simulink model "MecanumAndObjectTrackingModel"  (R2019b)
settings: Solver=VariableStepAuto  StartTime=0.0  StopTime=10.0  RelTol=1e-3
undefined symbols (not defined in the file): objLabel, objX, objY, sampleTime, targetLabel
libraries: mobileRoboticsLib x8
settings Model: Creator=spenc  LastModifiedBy=spenc

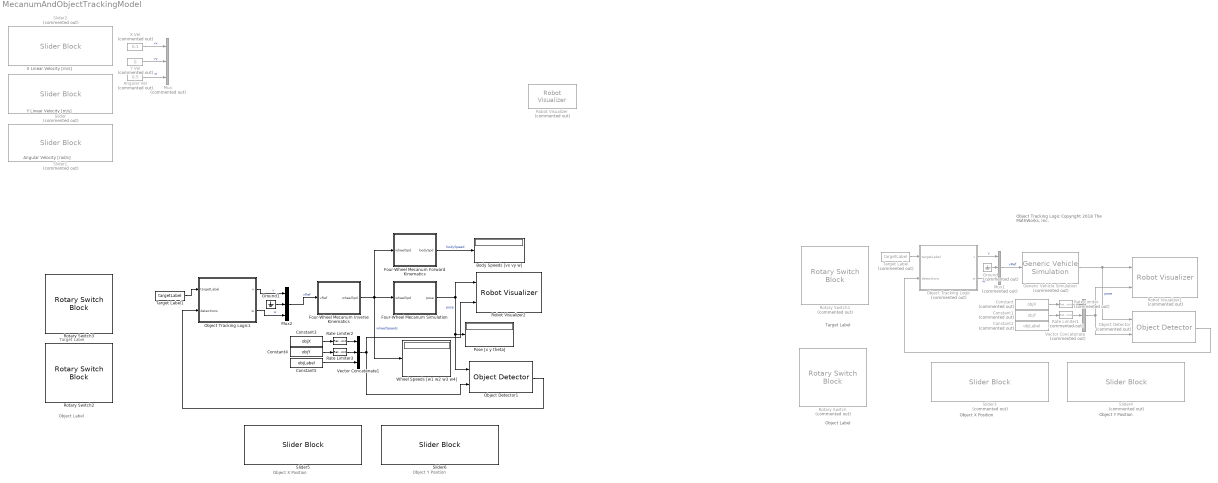
== system MecanumAndObjectTrackingModel ==
  note: Y Linear Velocity [m/s]
  note: Angular Velocity [rad/s]
  note: X Linear Velocity [m/s]
  note: Object X Position
  note: Object Tracking Logic
      |
      | Copyright 2018 The MathWorks, Inc.
  note: Target Label
  note: Object Y Position
  note: Object Label
  note: Object Label
  note: Target Label
  note: Object Y Position
  note: Object X Position
  Angular Vel : Constant  Commented=on  Value=0.5
  Body Speeds [vx vy w] : Display
  Constant : Constant  Commented=on  Value=objX
  Constant1 : Constant  Commented=on  Value=objY
  Constant2 : Constant  Commented=on  Value=objLabel
  Constant3 : Constant  Value=objX
  Constant4 : Constant  Value=objY
  Constant5 : Constant  Value=objLabel
  Four-Wheel Mecanum Forward Kinematics : Subsystem  AncestorBlock=mobileRoboticsLib/Kinematic Models/Four-Wheel Mecanum/Four-Wheel Mecanum Forward Kinematics  mask(Four-Wheel Mecanum Forward Kinematics){wheelRadius=0.1, wheelBase=0.535, wheelTrack=0.459}
      mask prompts: wheelRadius "Wheel Radius [m]"; wheelBase "Wheelbase [m]"; wheelTrack "Track [m]"
      mask help:
      | Calculates the forward kinematics for a four-wheeled vehicle with Mecanum wheels.
      |
      | Input: Wheel speeds [w1; w2; w3; w4] (rad/s)
      |
      | Output: Vehicle velocities [vx; vy; w] in body coordinates (m/s, m/s, and rad/s)
      mask Help: web('matlab:edit mrsDocFourWheelMecanum')
  Four-Wheel Mecanum Inverse Kinematics : Subsystem  AncestorBlock=mobileRoboticsLib/Kinematic Models/Four-Wheel Mecanum/Four-Wheel Mecanum Inverse Kinematics  mask(Four-Wheel Mecanum Inverse Kinematics){wheelRadius=0.1, wheelBase=0.535, wheelTrack=0.459}
      mask prompts: wheelRadius "Wheel Radius [m]"; wheelBase "Wheelbase [m]"; wheelTrack "Track [m]"
      mask help:
      | Calculates the inverse kinematics for a four-wheeled vehicle with Mecanum wheels.
      |
      | Input: Vehicle velocities [vx; vy; w] in body coordinates (m/s, m/s, and rad/s)
      |
      | Output: Wheel speeds [w1; w2; w3; w4] (rad/s)
      mask Help: web('matlab:edit mrsDocFourWheelMecanum')
  Four-Wheel Mecanum Simulation : Subsystem  AncestorBlock=mobileRoboticsLib/Kinematic Models/Four-Wheel Mecanum/Four-Wheel Mecanum Simulation  mask(Four-Wheel Mecanum Simulation){wheelRadius=0.1, wheelBase=0.535, wheelTrack=0.459, initX=0, initY=0, initAngle=0, Ts=0.05}
      mask prompts: wheelRadius "Wheel Radius [m]"; wheelBase "Wheelbase [m]"; wheelTrack "Track [m]"; initX "Initial X Position [m]"; initY "Initial Y Position [m]"; initAngle "Initial Angle [rad]"; Ts "Sample Time"
      mask help:
      | Simulates the kinematics of a four-wheeled vehicle with Mecanum wheels, from a specified initial pose.
      |
      | Input: Wheel speeds [w1; w2; w3; w4] (rad/s)
      |
      | Output: Pose [x; y; theta], in m, m, and rad
      |
      | Set the Sample Time parameter to 0 for continuous-time simulation, or a positive number for discrete-time simulation.
      mask Help: web('matlab:edit mrsDocFourWheelMecanum')
      mask Callback Ts:
      | Ts = evalin('base',get_param(gcb,'Ts'));
      | blk = [gcb '/Generic Robot Simulation/Velocity Integrator'];
      | if Ts > 0
      |     set_param(blk,'OverrideUsingVariant','mode==2');
      | else
      |     set_param(blk,'OverrideUsingVariant','mode==1');
      | end
  Generic Vehicle Simulation : mobileRoboticsLib/Utilities/Generic Vehicle Simulation  Commented=on  initX=2  initY=3  initAngle=0  Ts=sampleTime
      settings: SourceProductName=Mobile Robotics Simulation Library
  Ground : Ground  Commented=on
  Ground1 : Ground
  Mux : Mux  Commented=on  Inputs=3
  Mux1 : Mux  Commented=on  Inputs=3
  Mux2 : Mux  Inputs=3
  Object Detector : mobileRoboticsLib/Environments/Object Detector  Commented=on  mapName=map  sensorOffset=objDetectorOffset  sensorAngle=objDetectorAngle  fieldOfView=objDetectorFOV  maxRange=objDetectorRange  maxDetections=objDetectorMaxHits  sampleTime=-1
      settings: SourceProductName=Ground Vehicles Library
  Object Detector1 : mobileRoboticsLib/Environments/Object Detector  mapName=map  sensorOffset=[0,0]  sensorAngle=0  fieldOfView=pi/4  maxRange=5  maxDetections=3  sampleTime=0.05
      settings: SourceProductName=Ground Vehicles Library
  Object Tracking Logic : Stateflow chart  Commented=on  TreatAsAtomicUnit=on
  Object Tracking Logic1 : Stateflow chart  TreatAsAtomicUnit=on
  Pose [x y theta] : Display
  Rate Limiter : RateLimiter  Commented=on  SampleTimeMode=inherited  InitialCondition=objX
  Rate Limiter1 : RateLimiter  Commented=on  SampleTimeMode=inherited  InitialCondition=objX
  Rate Limiter2 : RateLimiter  SampleTimeMode=inherited  InitialCondition=objX
  Rate Limiter3 : RateLimiter  SampleTimeMode=inherited  InitialCondition=objX
  Robot Visualizer : mobileRoboticsLib/Environments/Robot Visualizer  Priority=99  Commented=on  robotRadius=0  showTrajectory=on  hasWaypoints=off  hasLidar=off  sensorOffset=[ 0 0 ]  scanAngles=scanAngles  hasObjDetector=off  objDetectorOffset=[ 0, 0 ]  objDetectorAngle=0  objDetectorFOV=pi/4  objDetectorMaxRange=5  objectColors=[ 1, 0, 0; 0, 1, 0; 0, 0, 1 ]  objectMarkers=s
      settings: SourceProductName=Ground Vehicles Library
  Robot Visualizer1 : mobileRoboticsLib/Environments/Robot Visualizer  Priority=99  Commented=on  robotRadius=0  mapName=map  showTrajectory=on  hasWaypoints=off  hasLidar=off  sensorOffset=[ 0 0 ]  scanAngles=0  hasObjDetector=on  objDetectorOffset=objDetectorOffset  objDetectorAngle=objDetectorAngle  objDetectorFOV=objDetectorFOV  objDetectorMaxRange=objDetectorRange  objectColors=objDetectorColors  objectMarkers=s
      settings: SourceProductName=Ground Vehicles Library
  Robot Visualizer2 : mobileRoboticsLib/Environments/Robot Visualizer  Priority=99  robotRadius=0.5  mapName=map  showTrajectory=on  hasWaypoints=off  hasLidar=off  sensorOffset=[ 0 0 ]  scanAngles=0  hasObjDetector=on  objDetectorOffset=[0,0]  objDetectorAngle=[-pi/4,0,pi/4]  objDetectorFOV=pi/4  objDetectorMaxRange=5  objectColors=eye(3,3)  objectMarkers=s
      settings: SourceProductName=Ground Vehicles Library
  Rotary Switch : RotarySwitchBlock  Commented=on  LabelPosition=Hide
      settings: Values={{'RED', 'GREEN', 'BLUE'}, [1 2 3]}
  Rotary Switch1 : RotarySwitchBlock  Commented=on  LabelPosition=Hide
      settings: Values={{'RED', 'GREEN', 'BLUE'}, [1 2 3]}
  Rotary Switch2 : RotarySwitchBlock  LabelPosition=Hide
      settings: Values={{'RED', 'GREEN', 'BLUE'}, [1 2 3]}
  Rotary Switch3 : RotarySwitchBlock  LabelPosition=Hide
      settings: Values={{'RED', 'GREEN', 'BLUE'}, [1 2 3]}
  Slider : SliderBlock  Commented=on  ScaleMin=-1  ScaleMax=1  TickInterval=0.25
  Slider1 : SliderBlock  Commented=on  ScaleMin=-1.5  ScaleMax=1.5
  Slider2 : SliderBlock  Commented=on  ScaleMin=-1  ScaleMax=1  TickInterval=0.25
  Slider3 : SliderBlock  Commented=on  ScaleMax=13
  Slider4 : SliderBlock  Commented=on  ScaleMax=13
  Slider5 : SliderBlock  ScaleMax=13
  Slider6 : SliderBlock  ScaleMax=13
  Target Label : Constant  Commented=on  Value=targetLabel
  Target Label1 : Constant  Value=targetLabel
  Vector Concatenate : Concatenate  Commented=on  NumInputs=3  Mode=Multidimensional array  ConcatenateDimension=2
  Vector Concatenate1 : Concatenate  NumInputs=3  Mode=Multidimensional array  ConcatenateDimension=2
  Wheel Speeds [w1 w2 w3 w4] : Display
  X Vel : Constant  Commented=on  Value=0.1
  Y Vel : Constant  Commented=on  Value=0
  wires:
  Y Vel/1 -> Mux/2  "vy"
  Four-Wheel Mecanum Forward Kinematics/1(bodySpd) -> Body Speeds [vx vy w]/1  "bodySpeed"
  Four-Wheel Mecanum Simulation/1(pose) -> Robot Visualizer2/1, Object Detector1/1, Pose [x y theta]/1  "pose"
  Four-Wheel Mecanum Inverse Kinematics/1(wheelSpd) -> Four-Wheel Mecanum Forward Kinematics/1(wheelSpd), Four-Wheel Mecanum Simulation/1(wheelSpd), Wheel Speeds [w1 w2 w3 w4]/1  "wheelSpeeds"
  Angular Vel/1 -> Mux/3  "w"
  X Vel/1 -> Mux/1  "vx"
  Ground/1 -> Mux1/2
  Rate Limiter1/1 -> Vector Concatenate/2
  Target Label/1 -> Object Tracking Logic/1(targetLabel)
  Rate Limiter/1 -> Vector Concatenate/1
  Generic Vehicle Simulation/1 -> Object Detector/1, Robot Visualizer1/1  "pose"
  Object Tracking Logic/2(w) -> Mux1/3  "w"
  Vector Concatenate/1 -> Object Detector/2, Robot Visualizer1/2
  Object Tracking Logic/1(v) -> Mux1/1  "v"
  Object Detector/1 -> Object Tracking Logic/2(detections)
  Constant/1 -> Rate Limiter/1
  Mux1/1 -> Generic Vehicle Simulation/1  "vRef"
  Constant2/1 -> Vector Concatenate/3
  Constant1/1 -> Rate Limiter1/1
  Mux2/1 -> Four-Wheel Mecanum Inverse Kinematics/1(vRef)  "vRef"
  Object Detector1/1 -> Object Tracking Logic1/2(detections)
  Object Tracking Logic1/2(w) -> Mux2/3  "w"
  Target Label1/1 -> Object Tracking Logic1/1(targetLabel)
  Ground1/1 -> Mux2/2
  Object Tracking Logic1/1(v) -> Mux2/1  "v"
  Constant4/1 -> Rate Limiter3/1
  Constant5/1 -> Vector Concatenate1/3
  Constant3/1 -> Rate Limiter2/1
  Rate Limiter2/1 -> Vector Concatenate1/1
  Rate Limiter3/1 -> Vector Concatenate1/2
  Vector Concatenate1/1 -> Object Detector1/2, Robot Visualizer2/2

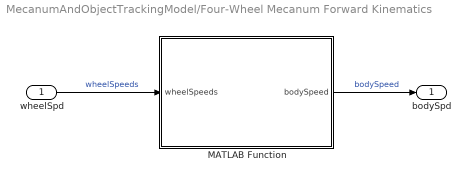
== system MecanumAndObjectTrackingModel/Four-Wheel Mecanum Forward Kinematics ==
  wheelSpd : Inport
  MATLAB Function : MATLAB Function  TreatAsAtomicUnit=on
  bodySpd : Outport  VectorParamsAs1DForOutWhenUnconnected=off
  wires:
  wheelSpd/1 -> MATLAB Function/1(wheelSpeeds)  "wheelSpeeds"
  MATLAB Function/1(bodySpeed) -> bodySpd/1  "bodySpeed"

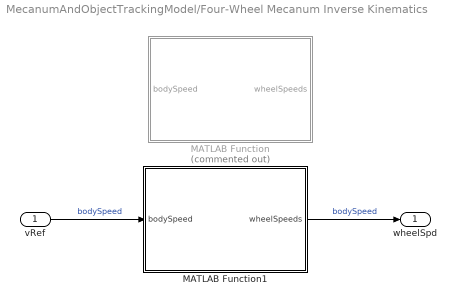
== system MecanumAndObjectTrackingModel/Four-Wheel Mecanum Inverse Kinematics ==
  vRef : Inport
  MATLAB Function : MATLAB Function  Commented=on  TreatAsAtomicUnit=on
  MATLAB Function1 : MATLAB Function  TreatAsAtomicUnit=on
  wheelSpd : Outport  VectorParamsAs1DForOutWhenUnconnected=off
  wires:
  vRef/1 -> MATLAB Function1/1(bodySpeed)  "bodySpeed"
  MATLAB Function1/1(wheelSpeeds) -> wheelSpd/1  "bodySpeed"

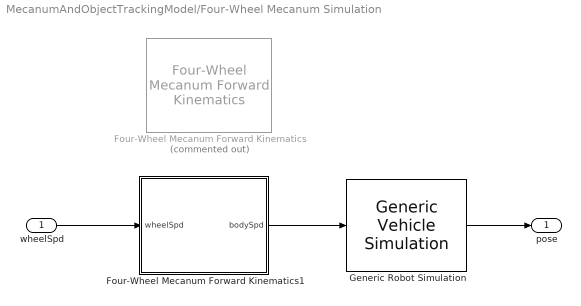
== system MecanumAndObjectTrackingModel/Four-Wheel Mecanum Simulation ==
  wheelSpd : Inport
  Four-Wheel Mecanum Forward Kinematics : mobileRoboticsLib/Kinematic Models/Four-Wheel Mecanum/Four-Wheel Mecanum Forward Kinematics  Commented=on  wheelRadius=0.1  wheelBase=0.535  wheelTrack=0.459
      settings: SourceProductName=Mobile Robotics Simulation Toolbox
  Four-Wheel Mecanum Forward Kinematics1 : Subsystem  AncestorBlock=mobileRoboticsLib/Kinematic Models/Four-Wheel Mecanum/Four-Wheel Mecanum Forward Kinematics  mask(Four-Wheel Mecanum Forward Kinematics){wheelRadius=0.1, wheelBase=0.535, wheelTrack=0.459}
      mask prompts: wheelRadius "Wheel Radius [m]"; wheelBase "Wheelbase [m]"; wheelTrack "Track [m]"
      mask help:
      | Calculates the forward kinematics for a four-wheeled vehicle with Mecanum wheels.
      |
      | Input: Wheel speeds [w1; w2; w3; w4] (rad/s)
      |
      | Output: Vehicle velocities [vx; vy; w] in body coordinates (m/s, m/s, and rad/s)
      mask Help: web('matlab:edit mrsDocFourWheelMecanum')
  Generic Robot Simulation : mobileRoboticsLib/Utilities/Generic Vehicle Simulation  initX=initX  initY=initY  initAngle=initAngle  Ts=Ts
      settings: SourceProductName=Mobile Robotics Simulation Toolbox
  pose : Outport  VectorParamsAs1DForOutWhenUnconnected=off
  wires:
  Generic Robot Simulation/1 -> pose/1
  wheelSpd/1 -> Four-Wheel Mecanum Forward Kinematics1/1(wheelSpd)
  Four-Wheel Mecanum Forward Kinematics1/1(bodySpd) -> Generic Robot Simulation/1

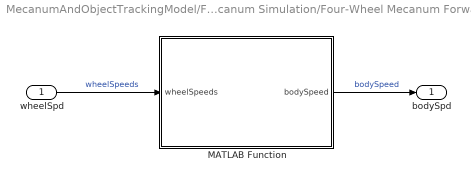
== system MecanumAndObjectTrackingModel/Four-Wheel Mecanum Simulation/Four-Wheel Mecanum Forward Kinematics1 ==
  wheelSpd : Inport
  MATLAB Function : MATLAB Function  TreatAsAtomicUnit=on
  bodySpd : Outport  VectorParamsAs1DForOutWhenUnconnected=off
  wires:
  MATLAB Function/1(bodySpeed) -> bodySpd/1  "bodySpeed"
  wheelSpd/1 -> MATLAB Function/1(wheelSpeeds)  "wheelSpeeds"

== stateflow chart MecanumAndObjectTrackingModel/Object Tracking Logic1 ==
  state TrackObject
    entry, during:
    [range,angle,valid] = findValidObject(targetLabel);
    if valid
    count = 0;
    else
    count = count + 1;
    end
    (default) -> (junction 20)
    TrackObject -> (junction 20) [order 1]
    (junction 20) -> (junction 24) [order 1] : % Set angular speed if
        | % angle outside deadband
        | [abs(angle) > pi/24]
    (junction 20) -> (junction 30) [order 2] : {w = 0;}
    (junction 24) -> (junction 49) : % Proportional
        | % control
        | {w = 1.5*angle;}
    (junction 49) -> (junction 30)
    (junction 30) -> (junction 54)
    (junction 54) -> (junction 56) [order 1] : % Go forward if object is far
        | [range > 1]
    (junction 54) -> (junction 60) [order 2] : {v = 0;}
    (junction 56) -> (junction 58) : {v = 0.5;}
    (junction 58) -> (junction 60)
  state SeekObject
    entry:
    v = 0;
    w = 1;
  (default) -> TrackObject : {
      | count = 0;
      | range = 0;
      | angle = 0;
      | }
  TrackObject -> SeekObject [order 1] : [count > 20]
  SeekObject -> TrackObject : [~isempty(detections)]
  data: dist function_output; ang function_output; flag function_output; label function_input; targetLabel input; detections input size=[objDetectorMaxHits,3]; v output; w output; angle local; range local; count local; valid local
  function [dist,ang,flag] = findValidObject(label):
    | function [dist,ang,flag] = findValidObject(label)
    | % Finds the distance (dist) and angle (ang) of the nearest valid
    | % object detected. If an object is found, the (flag) output is true.
    | 
    | % Initialize
    | flag = false;
    | dist = 0;
    | ang = 0;
    | 
    | if ~isempty(detections)
    |     % Loop through all detections
    |     for idx = 1:size(detections,1)
    |         % If a detection matching the target label is found, 
    |         % return it and set the valid flag to true.
    |         if detections(idx,3) == label
    |             dist = detections(idx,1);
    |             ang  = detections(idx,2);
    |             flag = true;
    |             return; 
    |         end
    |     end
    | end

== matlab function MecanumAndObjectTrackingModel/Four-Wheel Mecanum Inverse Kinematics/MATLAB Function1 ==
  data: bodySpeed input; wheelRadius parameter; wheelSpeeds output; wheelBase parameter; wheelTrack parameter
function wheelSpeeds = fourWheelMecanumInvKin(bodySpeed,wheelRadius,wheelBase,wheelTrack)
    
    % Initialize FourWheelMecanum object
    persistent robot
    if isempty(robot)
        robot = FourWheelMecanum_toolbox(wheelRadius,wheelBase,wheelTrack);
    end
    
    % Run object's inverse kinematics method
    wheelSpeeds = inverseKinematics(robot,bodySpeed);

end

== stateflow chart MecanumAndObjectTrackingModel/Object Tracking Logic ==
  state TrackObject
    entry, during:
    [range,angle,valid] = findValidObject(targetLabel);
    if valid
    count = 0;
    else
    count = count + 1;
    end
    (default) -> (junction 20)
    TrackObject -> (junction 20) [order 1]
    (junction 20) -> (junction 24) [order 1] : % Set angular speed if
        | % angle outside deadband
        | [abs(angle) > pi/24]
    (junction 20) -> (junction 30) [order 2] : {w = 0;}
    (junction 24) -> (junction 49) : % Proportional
        | % control
        | {w = 1.5*angle;}
    (junction 49) -> (junction 30)
    (junction 30) -> (junction 54)
    (junction 54) -> (junction 56) [order 1] : % Go forward if object is far
        | [range > 1]
    (junction 54) -> (junction 60) [order 2] : {v = 0;}
    (junction 56) -> (junction 58) : {v = 0.5;}
    (junction 58) -> (junction 60)
  state SeekObject
    entry:
    v = 0;
    w = 1;
  (default) -> TrackObject : {
      | count = 0;
      | range = 0;
      | angle = 0;
      | }
  TrackObject -> SeekObject [order 1] : [count > 20]
  SeekObject -> TrackObject : [~isempty(detections)]
  data: dist function_output; ang function_output; flag function_output; label function_input; targetLabel input; detections input size=[objDetectorMaxHits,3]; v output; w output; angle local; range local; count local; valid local
  function [dist,ang,flag] = findValidObject(label):
    | function [dist,ang,flag] = findValidObject(label)
    | % Finds the distance (dist) and angle (ang) of the nearest valid
    | % object detected. If an object is found, the (flag) output is true.
    | 
    | % Initialize
    | flag = false;
    | dist = 0;
    | ang = 0;
    | 
    | if ~isempty(detections)
    |     % Loop through all detections
    |     for idx = 1:size(detections,1)
    |         % If a detection matching the target label is found, 
    |         % return it and set the valid flag to true.
    |         if detections(idx,3) == label
    |             dist = detections(idx,1);
    |             ang  = detections(idx,2);
    |             flag = true;
    |             return; 
    |         end
    |     end
    | end

== matlab function MecanumAndObjectTrackingModel/Four-Wheel Mecanum Simulation/Four-Wheel Mecanum Forward Kinematics1/MATLAB Function ==
  settings: updateMethod=DISCRETE
  data: wheelSpeeds input; bodySpeed output; wheelRadius parameter; wheelBase parameter; wheelTrack parameter
function bodySpeed = fourWheelMecanumFwdKin(wheelSpeeds,wheelRadius,wheelBase,wheelTrack)
    
    % Initialize FourWheelMecanum object
    persistent robot
    if isempty(robot)
        robot = FourWheelMecanum_toolbox(wheelRadius,wheelBase,wheelTrack);
    end
    
    % Run object's forward kinematics method
    bodySpeed = forwardKinematics(robot,wheelSpeeds);

end

== matlab function MecanumAndObjectTrackingModel/Four-Wheel Mecanum Forward Kinematics/MATLAB Function ==
  settings: updateMethod=DISCRETE
  data: wheelSpeeds input; bodySpeed output; wheelRadius parameter; wheelBase parameter; wheelTrack parameter
function bodySpeed = fourWheelMecanumFwdKin(wheelSpeeds,wheelRadius,wheelBase,wheelTrack)
    
    % Initialize FourWheelMecanum object
%% 
    persistent robot
    if isempty(robot)
        robot = FourWheelMecanum(wheelRadius,wheelBase,wheelTrack);
    end
    
    % Run object's forward kinematics method
    bodySpeed = forwardKinematics(robot,wheelSpeeds);

end

== matlab function MecanumAndObjectTrackingModel/Four-Wheel Mecanum Inverse Kinematics/MATLAB Function ==
  data: bodySpeed input; wheelRadius parameter; wheelSpeeds output; wheelBase parameter; wheelTrack parameter
function wheelSpeeds = fourWheelMecanumInvKin(bodySpeed,wheelRadius,wheelBase,wheelTrack)
    
    % Initialize FourWheelMecanum object
    persistent robot
    if isempty(robot)
        robot = FourWheelMecanum(wheelRadius,wheelBase,wheelTrack);
    end
    
    % Run object's inverse kinematics method
    wheelSpeeds = inverseKinematics(robot,bodySpeed);

end
